simulink model "asn_4_bb_acs"  (R2023b)
settings: Solver=VariableStepAuto  StartTime=0.0  StopTime=50  RelTol=1e-2  AbsTol=1e-2
values from neighbouring files (symbols this model uses):
  C_i = eul2rotm(eul_i, 'ZYX')    [asn_4_bb_script.m]
  H_M = [0 dz -dy 0 dz -dy 0 -dz dy 0 -dz dy ... (first row only)    [asn_4_bb_script.m]
  K_d = J*2*zeta*w_n    (= 70)    [asn_4_bb_script.m]
  K_p = 2*J*w_n^2    (= 50)    [asn_4_bb_script.m]
  q_i = eul2quat(deg2rad([42 -16 23]), 'ZYX')    [asn_4_bb_script.m]
  u_a = 50    [asn_4_bb_script.m]
  w_i = [0;0;0]    [asn_4_bb_script.m]
undefined symbols (not defined in the file or in its folder): C_b_LVLH_i, eps_b_ECI_i, eps_b_LVLH_i, eta_b_ECI_i, eta_b_LVLH_i, phi_b_ECI_i, phi_b_LVLH_i, psi_b_ECEI_i, psi_b_LVLH_i, R_i, theta_b_ECI_i, theta_b_LVLH_i, V_i
libraries: matrix_library x1
settings Model: SimulationMode=accelerator  Creator=mikey  LastModifiedBy=mikey

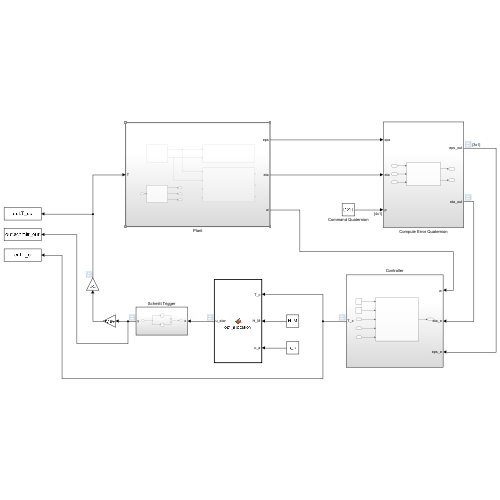
[thumbnail: Simulink's stored preview of the top-level diagram]
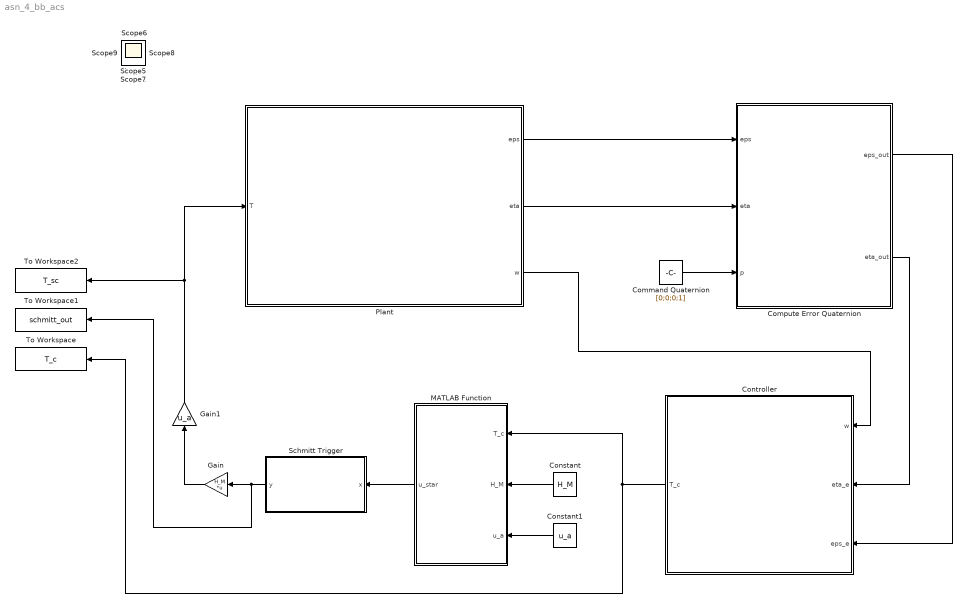
== system asn_4_bb_acs ==
  Command Quaternion : Constant  Value=[0;0;0;1]
  Compute Error Quaternion : Subsystem
  Constant : Constant  Value=H_M
  Constant1 : Constant  Value=u_a
  Controller : Subsystem
  Gain : Gain  Gain=H_M  Multiplication=Matrix(K*u) (u vector)
  Gain1 : Gain  Gain=u_a
  MATLAB Function : MATLAB Function  TreatAsAtomicUnit=on
  Plant : Subsystem
  Schmitt Trigger : Subsystem
  To Workspace : ToWorkspace  VariableName=T_c  SaveFormat=Timeseries  SampleTime=-1
  To Workspace1 : ToWorkspace  VariableName=schmitt_out  SaveFormat=Timeseries  SampleTime=-1
  To Workspace2 : ToWorkspace  VariableName=T_sc  SaveFormat=Timeseries  SampleTime=-1
  Scope{,1..9} (10 alike) : Scope
  wires:
  Command Quaternion/1 -> Compute Error Quaternion/3(p)
  Compute Error Quaternion/1(eps_out) -> Controller/3(eps_e)
  Compute Error Quaternion/2(eta_out) -> Controller/2(eta_e)
  Plant/2(eta) -> Compute Error Quaternion/2(eta)
  Plant/1(eps) -> Compute Error Quaternion/1(eps)
  Plant/3(w) -> Controller/1(w)
  Constant/1 -> MATLAB Function/2(H_M)
  Constant1/1 -> MATLAB Function/3(u_a)
  Controller/1(T_c) -> MATLAB Function/1(T_c), To Workspace/1
  MATLAB Function/1(u_star) -> Schmitt Trigger/1(x)
  Schmitt Trigger/1(y) -> To Workspace1/1, Gain/1
  Gain/1 -> Gain1/1
  Gain1/1 -> Plant/1(T), To Workspace2/1

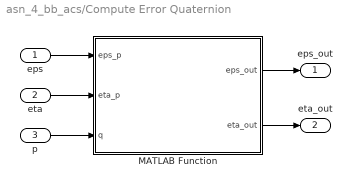
== system asn_4_bb_acs/Compute Error Quaternion ==
  eps : Inport
  eta : Inport  Port=2  PortDimensions=1
  p : Inport  Port=3  PortDimensions=[4,1]
  MATLAB Function : MATLAB Function  TreatAsAtomicUnit=on
  eps_out : Outport  PortDimensions=[3,1]
  eta_out : Outport  Port=2  PortDimensions=1
  wires:
  MATLAB Function/1(eps_out) -> eps_out/1
  p/1 -> MATLAB Function/3(q)
  eps/1 -> MATLAB Function/1(eps_p)
  eta/1 -> MATLAB Function/2(eta_p)
  MATLAB Function/2(eta_out) -> eta_out/1

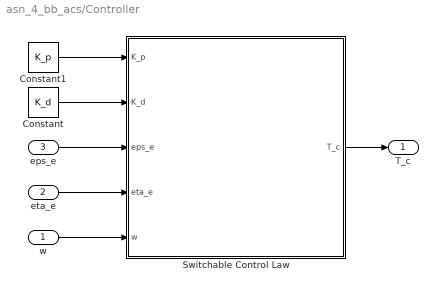
== system asn_4_bb_acs/Controller ==
  w : Inport
  eta_e : Inport  Port=2
  eps_e : Inport  Port=3
  Constant : Constant  Value=K_d
  Constant1 : Constant  Value=K_p
  Switchable Control Law : MATLAB Function  TreatAsAtomicUnit=on
  T_c : Outport
  wires:
  w/1 -> Switchable Control Law/5(w)
  Switchable Control Law/1(T_c) -> T_c/1
  eps_e/1 -> Switchable Control Law/3(eps_e)
  eta_e/1 -> Switchable Control Law/4(eta_e)
  Constant/1 -> Switchable Control Law/2(K_d)
  Constant1/1 -> Switchable Control Law/1(K_p)

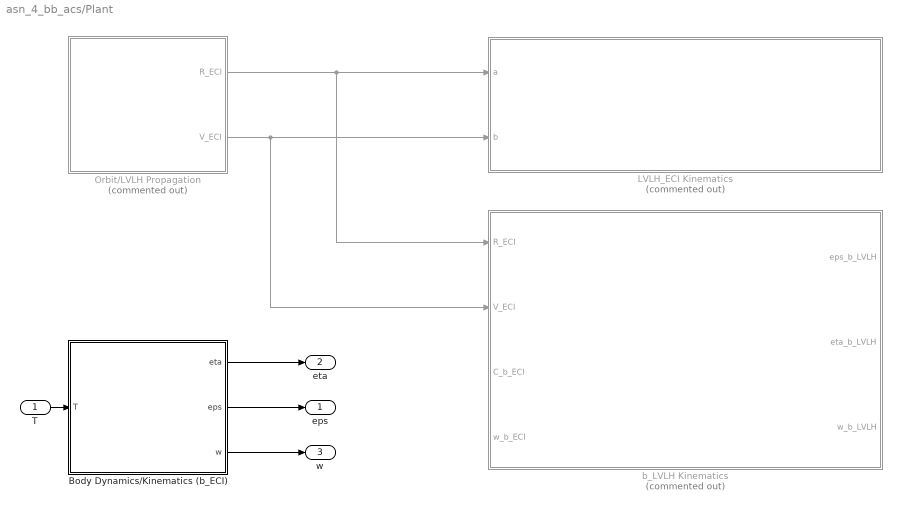
== system asn_4_bb_acs/Plant ==
  T : Inport
  Body Dynamics/Kinematics (b_ECI) : Subsystem
  LVLH_ECI Kinematics : Subsystem  Commented=on
  Orbit/LVLH Propagation : Subsystem  Commented=on
  b_LVLH Kinematics : Subsystem  Commented=on
  eps : Outport
  eta : Outport  Port=2
  w : Outport  Port=3
  wires:
  Orbit/LVLH Propagation/2(V_ECI) -> b_LVLH Kinematics/2(V_ECI), LVLH_ECI Kinematics/2(b)
  Orbit/LVLH Propagation/1(R_ECI) -> b_LVLH Kinematics/1(R_ECI), LVLH_ECI Kinematics/1(a)
  T/1 -> Body Dynamics/Kinematics (b_ECI)/1(T)
  Body Dynamics/Kinematics (b_ECI)/1(eta) -> eta/1
  Body Dynamics/Kinematics (b_ECI)/2(eps) -> eps/1
  Body Dynamics/Kinematics (b_ECI)/3(w) -> w/1

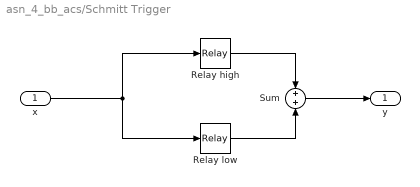
== system asn_4_bb_acs/Schmitt Trigger ==
  x : Inport
  Relay high : Relay  OnSwitchValue=0.002*ones(12,1)  OffSwitchValue=0.001*ones(12,1)  OnOutputValue=ones(12,1)  OffOutputValue=zeros(12,1)
  Relay low : Relay  OnSwitchValue=-0.001*ones(12,1)  OffSwitchValue=-0.002*ones(12,1)  OnOutputValue=zeros(12,1)  OffOutputValue=-ones(12,1)
  Sum : Sum  Inputs=+|+
  y : Outport
  wires:
  x/1 -> Relay high/1, Relay low/1
  Relay high/1 -> Sum/1
  Relay low/1 -> Sum/2
  Sum/1 -> y/1

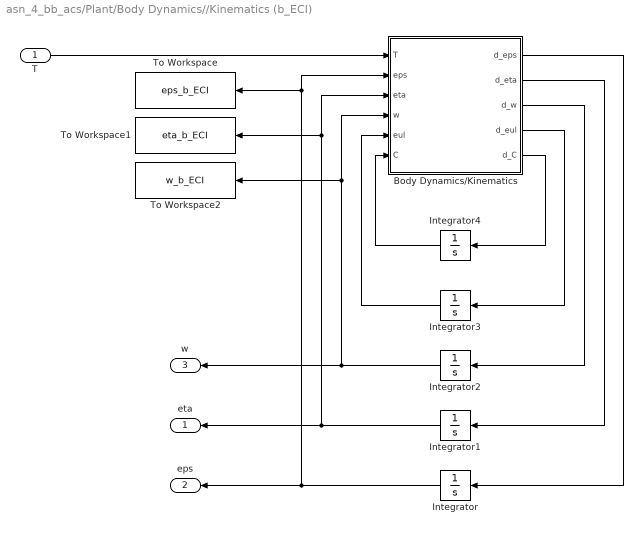
== system asn_4_bb_acs/Plant/Body Dynamics//Kinematics (b_ECI) ==
  T : Inport
  Body Dynamics/Kinematics : MATLAB Function  TreatAsAtomicUnit=on
  Integrator : Integrator  InitialCondition=q_i(1:3)'
  Integrator1 : Integrator  InitialCondition=q_i(4)
  Integrator2 : Integrator  InitialCondition=w_i
  Integrator3 : Integrator  InitialCondition=eul_i'
  Integrator4 : Integrator  InitialCondition=C_i
  To Workspace : ToWorkspace  VariableName=eps_b_ECI  SaveFormat=Timeseries  SampleTime=-1
      settings: Save2DSignal=2-D array (concatenate along first dimension)
  To Workspace1 : ToWorkspace  VariableName=eta_b_ECI  SaveFormat=Timeseries  SampleTime=-1
      settings: Save2DSignal=2-D array (concatenate along first dimension)
  To Workspace2 : ToWorkspace  VariableName=w_b_ECI  SaveFormat=Timeseries  SampleTime=-1
      settings: Save2DSignal=2-D array (concatenate along first dimension)
  eta : Outport
  eps : Outport  Port=2
  w : Outport  Port=3
  wires:
  Integrator1/1 -> eta/1, To Workspace1/1, Body Dynamics/Kinematics/3(eta)
  Body Dynamics/Kinematics/2(d_eta) -> Integrator1/1
  Body Dynamics/Kinematics/4(d_eul) -> Integrator3/1
  Integrator2/1 -> To Workspace2/1, Body Dynamics/Kinematics/4(w), w/1
  Body Dynamics/Kinematics/3(d_w) -> Integrator2/1
  Integrator3/1 -> Body Dynamics/Kinematics/5(eul)
  Integrator/1 -> Body Dynamics/Kinematics/2(eps), To Workspace/1, eps/1
  Body Dynamics/Kinematics/1(d_eps) -> Integrator/1
  Body Dynamics/Kinematics/5(d_C) -> Integrator4/1
  Integrator4/1 -> Body Dynamics/Kinematics/6(C)
  T/1 -> Body Dynamics/Kinematics/1(T)

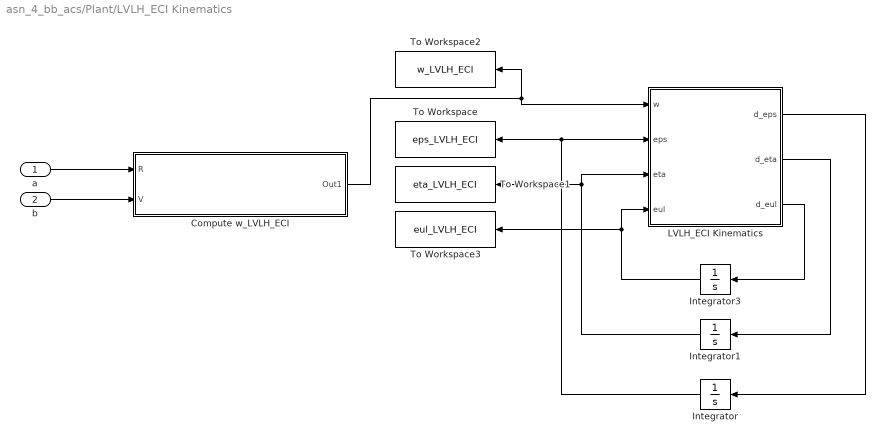
== system asn_4_bb_acs/Plant/LVLH_ECI Kinematics ==
  a : Inport
  b : Inport  Port=2
  Compute w_LVLH_ECI : Subsystem
  Integrator : Integrator  InitialCondition=eps_b_ECI_i
  Integrator1 : Integrator  InitialCondition=eta_b_ECI_i
  Integrator3 : Integrator  InitialCondition=[phi_b_ECI_i; theta_b_ECI_i; psi_b_ECEI_i]
  LVLH_ECI Kinematics : MATLAB Function  TreatAsAtomicUnit=on
  To Workspace : ToWorkspace  VariableName=eps_LVLH_ECI  SampleTime=-1
      settings: Save2DSignal=2-D array (concatenate along first dimension)
  To Workspace1 : ToWorkspace  VariableName=eta_LVLH_ECI  SampleTime=-1
      settings: Save2DSignal=2-D array (concatenate along first dimension)
  To Workspace2 : ToWorkspace  VariableName=w_LVLH_ECI  SampleTime=-1
      settings: Save2DSignal=2-D array (concatenate along first dimension)
  To Workspace3 : ToWorkspace  VariableName=eul_LVLH_ECI  SampleTime=-1
      settings: Save2DSignal=2-D array (concatenate along first dimension)
  wires:
  LVLH_ECI Kinematics/1(d_eps) -> Integrator/1
  LVLH_ECI Kinematics/3(d_eul) -> Integrator3/1
  Integrator1/1 -> To Workspace1/1, LVLH_ECI Kinematics/3(eta)
  Integrator3/1 -> LVLH_ECI Kinematics/4(eul), To Workspace3/1
  LVLH_ECI Kinematics/2(d_eta) -> Integrator1/1
  Integrator/1 -> LVLH_ECI Kinematics/2(eps), To Workspace/1
  Compute w_LVLH_ECI/1(Out1) -> LVLH_ECI Kinematics/1(w), To Workspace2/1
  a/1 -> Compute w_LVLH_ECI/1(R)
  b/1 -> Compute w_LVLH_ECI/2(V)

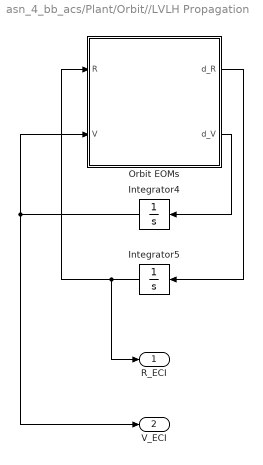
== system asn_4_bb_acs/Plant/Orbit//LVLH Propagation ==
  Integrator4 : Integrator  InitialCondition=V_i
  Integrator5 : Integrator  InitialCondition=R_i
  Orbit EOMs : MATLAB Function  TreatAsAtomicUnit=on
  R_ECI : Outport
  V_ECI : Outport  Port=2
  wires:
  Orbit EOMs/2(d_V) -> Integrator4/1
  Integrator4/1 -> V_ECI/1, Orbit EOMs/2(V)
  Orbit EOMs/1(d_R) -> Integrator5/1
  Integrator5/1 -> Orbit EOMs/1(R), R_ECI/1

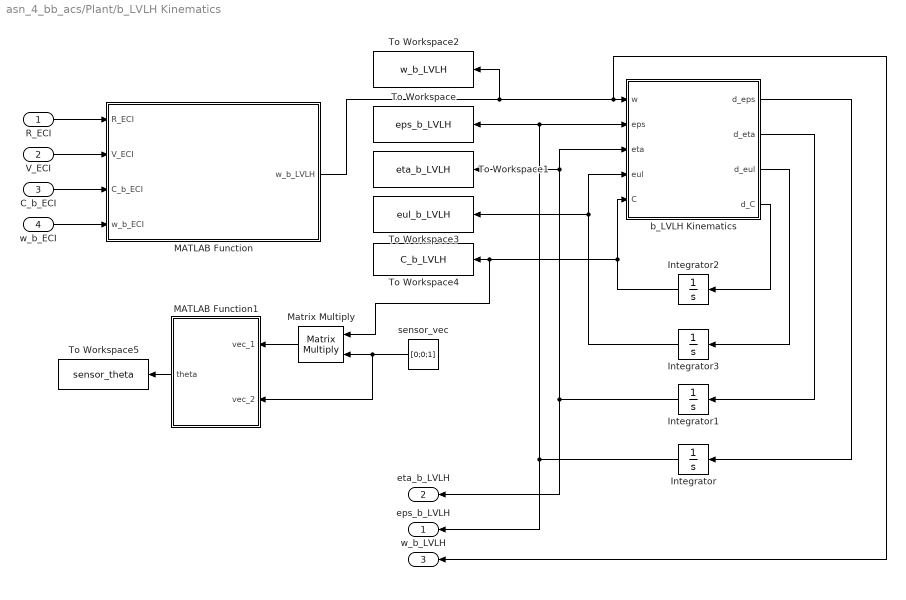
== system asn_4_bb_acs/Plant/b_LVLH Kinematics ==
  R_ECI : Inport
  V_ECI : Inport  Port=2
  C_b_ECI : Inport  Port=3
  w_b_ECI : Inport  Port=4
  Integrator : Integrator  InitialCondition=eps_b_LVLH_i
  Integrator1 : Integrator  InitialCondition=eta_b_LVLH_i
  Integrator2 : Integrator  InitialCondition=C_b_LVLH_i
  Integrator3 : Integrator  InitialCondition=[phi_b_LVLH_i;theta_b_LVLH_i;psi_b_LVLH_i]
  MATLAB Function : MATLAB Function  TreatAsAtomicUnit=on
  MATLAB Function1 : MATLAB Function  TreatAsAtomicUnit=on
  Matrix Multiply : Product  Multiplication=Matrix(*)
  To Workspace : ToWorkspace  VariableName=eps_b_LVLH  SampleTime=-1
      settings: Save2DSignal=2-D array (concatenate along first dimension)
  To Workspace1 : ToWorkspace  VariableName=eta_b_LVLH  SampleTime=-1
      settings: Save2DSignal=2-D array (concatenate along first dimension)
  To Workspace2 : ToWorkspace  VariableName=w_b_LVLH  SampleTime=-1
      settings: Save2DSignal=2-D array (concatenate along first dimension)
  To Workspace3 : ToWorkspace  VariableName=eul_b_LVLH  SampleTime=-1
      settings: Save2DSignal=2-D array (concatenate along first dimension)
  To Workspace4 : ToWorkspace  VariableName=C_b_LVLH  SampleTime=-1
  To Workspace5 : ToWorkspace  VariableName=sensor_theta  SampleTime=-1
      settings: Save2DSignal=2-D array (concatenate along first dimension)
  b_LVLH Kinematics : MATLAB Function  TreatAsAtomicUnit=on
  sensor_vec : Constant  Value=[0;0;1]
  eps_b_LVLH : Outport
  eta_b_LVLH : Outport  Port=2
  w_b_LVLH : Outport  Port=3
  wires:
  MATLAB Function/1(w_b_LVLH) -> w_b_LVLH/1, b_LVLH Kinematics/1(w), To Workspace2/1
  Integrator1/1 -> To Workspace1/1, b_LVLH Kinematics/3(eta), eta_b_LVLH/1
  b_LVLH Kinematics/3(d_eul) -> Integrator3/1
  Integrator/1 -> b_LVLH Kinematics/2(eps), To Workspace/1, eps_b_LVLH/1
  Integrator3/1 -> b_LVLH Kinematics/4(eul), To Workspace3/1
  V_ECI/1 -> MATLAB Function/2(V_ECI)
  b_LVLH Kinematics/1(d_eps) -> Integrator/1
  b_LVLH Kinematics/2(d_eta) -> Integrator1/1
  R_ECI/1 -> MATLAB Function/1(R_ECI)
  C_b_ECI/1 -> MATLAB Function/3(C_b_ECI)
  w_b_ECI/1 -> MATLAB Function/4(w_b_ECI)
  b_LVLH Kinematics/4(d_C) -> Integrator2/1
  Integrator2/1 -> b_LVLH Kinematics/5(C), Matrix Multiply/1, To Workspace4/1
  sensor_vec/1 -> MATLAB Function1/2(vec_2), Matrix Multiply/2
  Matrix Multiply/1 -> MATLAB Function1/1(vec_1)
  MATLAB Function1/1(theta) -> To Workspace5/1

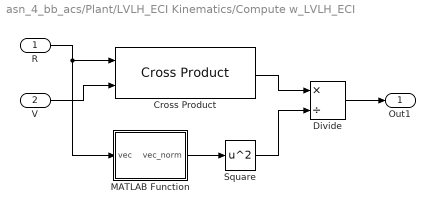
== system asn_4_bb_acs/Plant/LVLH_ECI Kinematics/Compute w_LVLH_ECI ==
  R : Inport
  V : Inport  Port=2
  Cross Product : matrix_library/Cross Product
  Divide : Product  Inputs=*/
  MATLAB Function : MATLAB Function  TreatAsAtomicUnit=on
  Square : Math  Operator=square
  Out1 : Outport
  wires:
  Divide/1 -> Out1/1
  Cross Product/1 -> Divide/1
  MATLAB Function/1(vec_norm) -> Square/1
  Square/1 -> Divide/2
  R/1 -> MATLAB Function/1(vec), Cross Product/1
  V/1 -> Cross Product/2

== matlab function asn_4_bb_acs/Controller/Switchable Control Law ==
  data: K_p input; K_d input; eps_e input; eta_e input; T_c output; w input
function T_c = FSFB(K_p, K_d, eps_e, eta_e, w)

    T_c = -K_p*eps_e - K_d*w;

== matlab function asn_4_bb_acs/MATLAB Function ==
  data: T_c input; u_star output; H_M input; u_a input
function u_star = opt_allocation(T_c, H_M, u_a)

f = ones(12,1);
Aeq = u_a*H_M;
beq = T_c;
lb = zeros(12,1);
ub = ones(12,1);

coder.extrinsic("linprog")
coder.extrinsic("optimoptions")

options = optimoptions('linprog','Display','none');
u_star = zeros(12,1);
u_star = linprog(f,[],[],Aeq,beq,lb,ub,options);

== matlab function asn_4_bb_acs/Plant/Orbit//LVLH Propagation/Orbit EOMs ==
  data: R input; d_R output; V input; d_V output
function [d_R,d_V] = orbitProp(R,V)

mu_earth = 398600;

x = R(1);
y = R(2);
z = R(3);

dx = V(1);
dy = V(2);
dz = V(3);

r = norm([x y z]);

ddx = (-mu_earth*x)/r^3;
ddy = (-mu_earth*y)/r^3;
ddz = (-mu_earth*z)/r^3;

d_R = [dx; dy; dz;];
d_V = [ddx; ddy; ddz];

end

== matlab function asn_4_bb_acs/Plant/Body Dynamics//Kinematics (b_ECI)/Body Dynamics//Kinematics ==
  data: T input; eps input; d_eps output; eta input; w input; eul input; d_eta output; d_w output; d_eul output; d_C output; C input
function [d_eps, d_eta, d_w, d_eul, d_C] = fcn(T, eps, eta, w, eul, C)

% satellite parameters
m = 750; % kg
J = m/12*diag([2 2 2]);

% cross matricies
w_cross = [0 -w(3) w(2);
           w(3) 0 -w(1);
          -w(2) w(1) 0]; % cross notation matrix


eps_cross = [0 -eps(3) eps(2);
             eps(3) 0 -eps(1); 
            -eps(2) eps(1) 0]; % cross matrix

% unpack other inputs
phi = eul(1);
theta = eul(2);
psi = eul(3);

eul_mat = [1, sin(phi)*tan(theta), cos(phi)*tan(theta); 0, cos(phi), -sin(phi); 0, sin(phi)*sec(theta), cos(phi)*sec(theta)];

% outputs
d_eps = 0.5*(eta*eye(3) + eps_cross)*w;

d_eta = -0.5*eps'*w;

d_w = J\(T - w_cross*J*w);

d_eul = eul_mat*w;

d_C = -w_cross*C;

== matlab function asn_4_bb_acs/Plant/b_LVLH Kinematics/MATLAB Function ==
  data: R_ECI input; w_b_LVLH output; V_ECI input; C_b_ECI input; w_b_ECI input
function w_b_LVLH = w_b_ECI_2_w_b_LVLH(R_ECI,V_ECI,C_b_ECI,w_b_ECI)

w_LVLH_ECI = cross(R_ECI,V_ECI)/(norm(R_ECI)^2);
w_b_LVLH = w_b_ECI - C_b_ECI*w_LVLH_ECI;

== matlab function asn_4_bb_acs/Plant/b_LVLH Kinematics/b_LVLH Kinematics ==
  data: w input; eps input; d_eps output; eta input; eul input; d_eta output; d_eul output; C input; d_C output
function [d_eps, d_eta, d_eul, d_C] = fcn(w, eps, eta, eul, C)

% satellite parameters
m = 3; % kg
J = m*1/12*[(0.1^2 + 0.3^2) 0 0;
            0 (0.1^2 + 0.3^2) 0;
            0 0 (0.1^2 + 0.1^2)]; % inertia tensor

% cross matricies
w_cross = [0 -w(3) w(2);
           w(3) 0 -w(1);
          -w(2) w(1) 0]; % cross notation matrix


eps_cross = [0 -eps(3) eps(2);
             eps(3) 0 -eps(1); 
            -eps(2) eps(1) 0]; % cross matrix

% unpack other inputs
phi = eul(1);
theta = eul(2);
psi = eul(3);

eul_mat = [1, sin(phi)*tan(theta), cos(phi)*tan(theta); 0, cos(phi), -sin(phi); 0, sin(phi)*sec(theta), cos(phi)*sec(theta)];

% outputs
d_eps = 0.5*(eta*eye(3) + eps_cross)*w;

d_eta = -0.5*eps'*w;

d_eul = eul_mat*w;

d_C = -w_cross*C;

== matlab function asn_4_bb_acs/Plant/LVLH_ECI Kinematics/LVLH_ECI Kinematics ==
  data: w input; eps input; d_eps output; eta input; eul input; d_eta output; d_eul output
function [d_eps, d_eta, d_eul] = fcn(w, eps, eta, eul)

% satellite parameters
m = 3; % kg
J = m*1/12*[(0.1^2 + 0.3^2) 0 0;
            0 (0.1^2 + 0.3^2) 0;
            0 0 (0.1^2 + 0.1^2)]; % inertia tensor

% cross matricies
w_cross = [0 -w(3) w(2);
           w(3) 0 -w(1);
          -w(2) w(1) 0]; % cross notation matrix


eps_cross = [0 -eps(3) eps(2);
             eps(3) 0 -eps(1); 
            -eps(2) eps(1) 0]; % cross matrix

% unpack other inputs
phi = eul(1);
theta = eul(2);
psi = eul(3);

eul_mat = [1, sin(phi)*tan(theta), cos(phi)*tan(theta); 0, cos(phi), -sin(phi); 0, sin(phi)*sec(theta), cos(phi)*sec(theta)];

% outputs
d_eps = 0.5*(eta*eye(3) + eps_cross)*w;

d_eta = -0.5*eps'*w;

d_eul = eul_mat*w;

== matlab function asn_4_bb_acs/Plant/LVLH_ECI Kinematics/Compute w_LVLH_ECI/MATLAB Function ==
  data: vec input; vec_norm output
function vec_norm = norm(vec)

vec_norm = norm(vec);

== matlab function asn_4_bb_acs/Plant/b_LVLH Kinematics/MATLAB Function1 ==
  data: vec_1 input; theta output; vec_2 input
function theta = angle_between(vec_1, vec_2)

theta = acos(dot(vec_1, vec_2)/(norm(vec_1)*norm(vec_2)));

== matlab function asn_4_bb_acs/Compute Error Quaternion/MATLAB Function ==
  data: eps_p input; eta_p input; eps_out output; q input; eta_out output
 function [eps_out,eta_out] = dotQuatMult(eps_p, eta_p, q)

eps_1 = eps_p(1);
eps_2 = eps_p(2);
eps_3 = eps_p(3);
eta = eta_p;

p_cir_mat =  [[eta, -eps_3, eps_2; eps_3, eta, -eps_1; -eps_2, eps_1, eta; -eps_1, -eps_2, -eps_3],[eps_p;eta_p]];

q_out = p_cir_mat*q;
eps_out = q_out(1:3);
eta_out = q_out(4);
